simulink model "vibration_fault_model"  (R2026a)
settings: Solver=VariableStepAuto  StopTime=300
undefined symbols (not defined in the file): engine

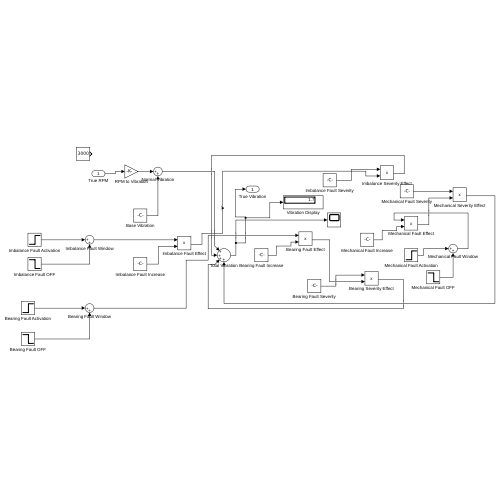
[thumbnail: Simulink's stored preview of the top-level diagram]
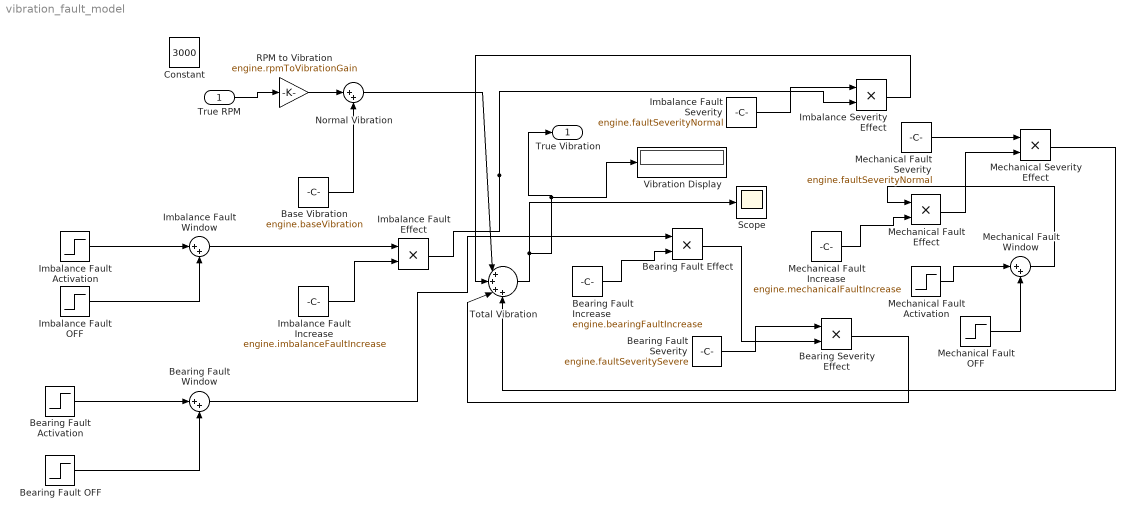
== system vibration_fault_model ==
  True RPM : Inport
  Base Vibration : Constant  Value=engine.baseVibration
  Bearing Fault Activation : Step  Time=180  SampleTime=0
  Bearing Fault Effect : Product
  Bearing Fault Increase : Constant  Value=engine.bearingFaultIncrease
  Bearing Fault OFF : Step  Time=240  FinalValue=-1  SampleTime=0
  Bearing Fault Severity : Constant  Value=engine.faultSeveritySevere
  Bearing Fault Window : Sum  Inputs=|++
  Bearing Severity Effect : Product
  Constant : Constant  Value=3000
  Imbalance Fault Activation : Step  Time=100  SampleTime=0
  Imbalance Fault Effect : Product
  Imbalance Fault Increase : Constant  Value=engine.imbalanceFaultIncrease
  Imbalance Fault OFF : Step  Time=180  FinalValue=-1  SampleTime=0
  Imbalance Fault Severity : Constant  Value=engine.faultSeverityNormal
  Imbalance Fault Window : Sum  Inputs=|++
  Imbalance Severity Effect : Product
  Mechanical Fault Activation : Step  Time=240  SampleTime=0
  Mechanical Fault Effect : Product
  Mechanical Fault Increase : Constant  Value=engine.mechanicalFaultIncrease
  Mechanical Fault OFF : Step  Time=300  FinalValue=-1  SampleTime=0
  Mechanical Fault Severity : Constant  Value=engine.faultSeverityNormal
  Mechanical Fault Window : Sum  Inputs=|++
  Mechanical Severity Effect : Product
  Normal Vibration : Sum  Inputs=|++
  RPM to Vibration : Gain  Gain=engine.rpmToVibrationGain
  Scope : Scope
      settings: ActiveDisplayYMinimum=1.5125  ActiveDisplayYMaximum=3.3875
  Total Vibration : Sum  Inputs=|++++
  Vibration Display : Display
  True Vibration : Outport
  wires:
  RPM to Vibration/1 -> Normal Vibration/1
  Base Vibration/1 -> Normal Vibration/2
  Imbalance Fault Increase/1 -> Imbalance Fault Effect/2
  Normal Vibration/1 -> Total Vibration/1
  Total Vibration/1 -> True Vibration/1, Vibration Display/1, Scope/1
  Bearing Fault Increase/1 -> Bearing Fault Effect/2
  Mechanical Fault Increase/1 -> Mechanical Fault Effect/2
  Imbalance Fault Effect/1 -> Imbalance Severity Effect/2
  Imbalance Fault Severity/1 -> Imbalance Severity Effect/1
  Imbalance Severity Effect/1 -> Total Vibration/2
  Bearing Fault Severity/1 -> Bearing Severity Effect/1
  Bearing Fault Effect/1 -> Bearing Severity Effect/2
  Bearing Severity Effect/1 -> Total Vibration/3
  Mechanical Fault Severity/1 -> Mechanical Severity Effect/1
  Mechanical Fault Effect/1 -> Mechanical Severity Effect/2
  Mechanical Severity Effect/1 -> Total Vibration/4
  Imbalance Fault Activation/1 -> Imbalance Fault Window/1
  Imbalance Fault OFF/1 -> Imbalance Fault Window/2
  Imbalance Fault Window/1 -> Imbalance Fault Effect/1
  Bearing Fault Activation/1 -> Bearing Fault Window/1
  Bearing Fault OFF/1 -> Bearing Fault Window/2
  Bearing Fault Window/1 -> Bearing Fault Effect/1
  Mechanical Fault Activation/1 -> Mechanical Fault Window/1
  Mechanical Fault OFF/1 -> Mechanical Fault Window/2
  Mechanical Fault Window/1 -> Mechanical Fault Effect/1
  True RPM/1 -> RPM to Vibration/1
